simulink model "c29_2"  (R2024a)
settings: Solver=FixedStepAuto  StartTime=0.0  StopTime=10.0  FixedStep=0.01  RelTol=1e-3
settings Model: Creator=17760  LastModifiedBy=17760

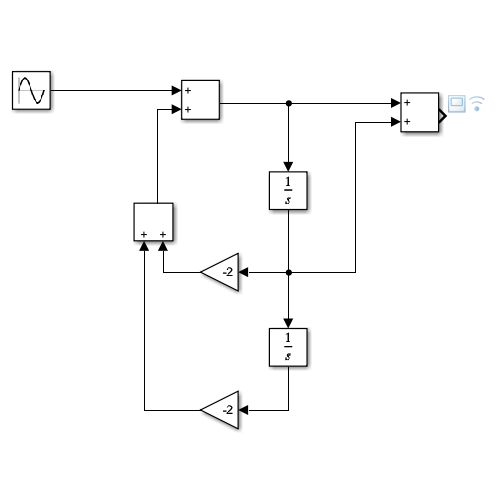
[thumbnail: Simulink's stored preview of the top-level diagram]
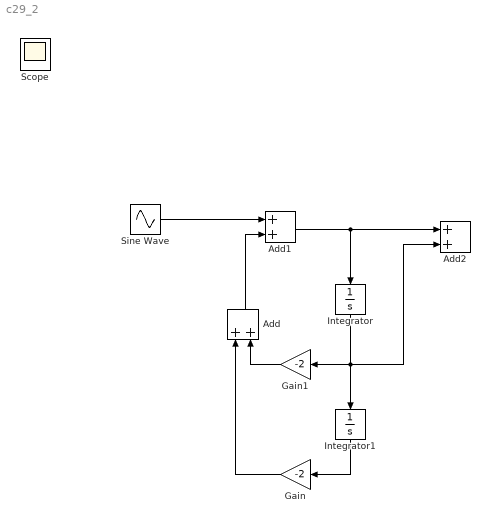
== system c29_2 ==
  Add : Sum
  Add1 : Sum
  Add2 : Sum
  Gain : Gain  Gain=-2
  Gain1 : Gain  Gain=-2
  Integrator : Integrator
  Integrator1 : Integrator
  Sine Wave : Sin  Frequency=3  SampleTime=0
  Scope : Scope
  wires:
  Add/1 -> Add1/2
  Sine Wave/1 -> Add1/1
  Add1/1 -> Integrator/1, Add2/1
  Integrator1/1 -> Gain/1
  Gain/1 -> Add/1
  Gain1/1 -> Add/2
  Integrator/1 -> Gain1/1, Integrator1/1, Add2/2
